simulink model "Part2"  (R2020b)
settings: Solver=VariableStepAuto  StartTime=0.0  StopTime=15  RelTol=1e-3
settings Model: Creator=abdullah  LastModifiedBy=abdullah

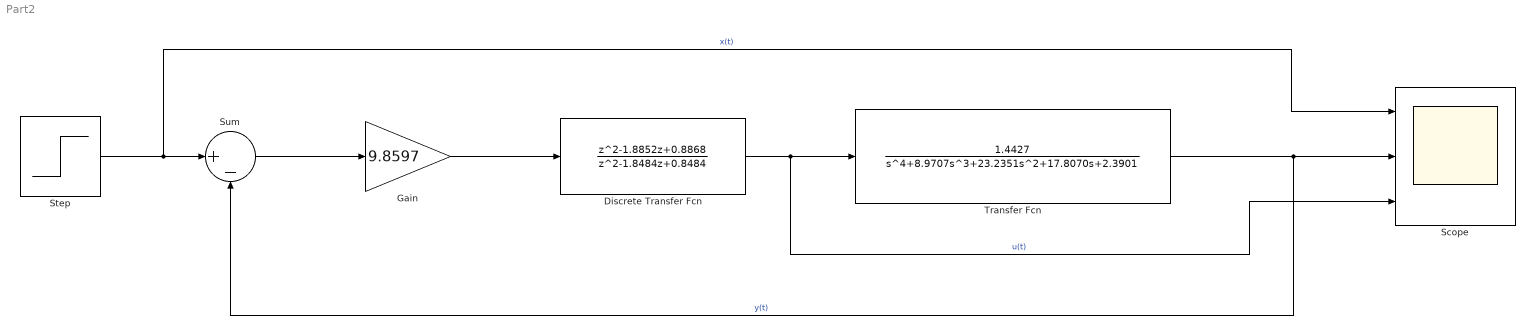
== system Part2 ==
  Discrete Transfer Fcn : DiscreteTransferFcn  Numerator="[1.0000   -1.8852    0.8868]"  Denominator="[1.0000   -1.8484    0.8484]"  SampleTime=0.1
  Gain : Gain  Gain=9.8597
  Scope : Scope  NumInputPorts=3
  Step : Step  SampleTime=0
  Sum : Sum  Inputs=|+-
  Transfer Fcn : TransferFcn  Numerator=[1.4427]  Denominator=[1 8.9707 23.2351 17.8070 2.3901]
  wires:
  Discrete Transfer Fcn/1 -> Scope/3, Transfer Fcn/1  "u(t)"
  Gain/1 -> Discrete Transfer Fcn/1
  Step/1 -> Scope/1, Sum/1  "x(t)"
  Sum/1 -> Gain/1
  Transfer Fcn/1 -> Sum/2, Scope/2  "y(t)"
